simulink model "TwoCellAMM"  (R2016b)
settings: Solver=VariableStepAuto  StartTime=0.0  StopTime=50.0  RelTol=1e-3
undefined symbols (not defined in the file or in its folder): k1, k2, m1, m2
libraries: simulink x1
settings Model: Creator=a1630459  LastModifiedBy=a1630459

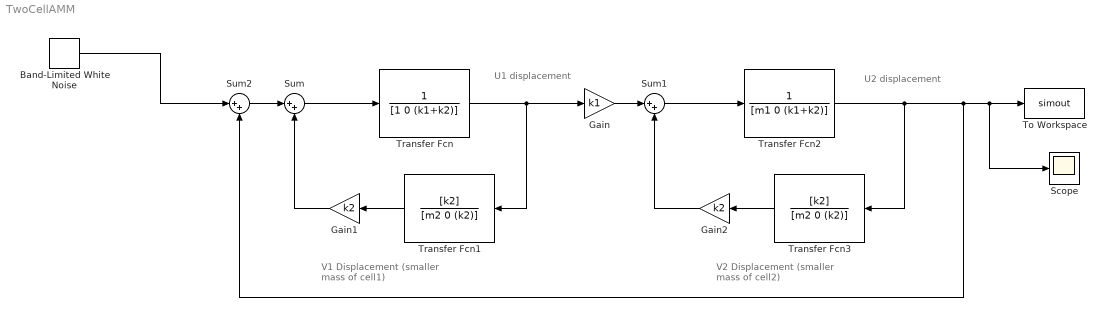
== system TwoCellAMM ==
  note: V1 Displacement
      | (smaller mass of cell1)
  note: U2 displacement
  note: U1 displacement
  note: V2 Displacement
      | (smaller mass of cell2)
  Band-Limited White Noise : simulink/Sources/Band-Limited White Noise  Cov=[0.1]  Ts=0.1  seed=[23341]
  Gain : Gain  Gain=k1
  Gain1 : Gain  Gain=k2
  Gain2 : Gain  Gain=k2
  Scope : Scope
  Sum : Sum  Inputs=|++
  Sum1 : Sum  Inputs=|++
  Sum2 : Sum  Inputs=|++
  To Workspace : ToWorkspace  VariableName=simout  SaveFormat=Timeseries  SampleTime=-1
  Transfer Fcn : TransferFcn  Denominator=[1 0 (k1+k2)]  ContinuousStateAttributes='displacement'
  Transfer Fcn1 : TransferFcn  Numerator=[k2]  Denominator=[m2 0 (k2)]  ContinuousStateAttributes='displacement'
  Transfer Fcn2 : TransferFcn  Denominator=[m1 0 (k1+k2)]  ContinuousStateAttributes='displacement'
  Transfer Fcn3 : TransferFcn  Numerator=[k2]  Denominator=[m2 0 (k2)]  ContinuousStateAttributes='displacement'
  wires:
  Sum/1 -> Transfer Fcn/1
  Gain/1 -> Sum1/1
  Transfer Fcn/1 -> Transfer Fcn1/1, Gain/1
  Transfer Fcn1/1 -> Gain1/1
  Gain1/1 -> Sum/2
  Sum2/1 -> Sum/1
  Sum1/1 -> Transfer Fcn2/1
  Gain2/1 -> Sum1/2
  Transfer Fcn3/1 -> Gain2/1
  Transfer Fcn2/1 -> Transfer Fcn3/1, Scope/1, To Workspace/1, Sum2/2
  Band-Limited White Noise/1 -> Sum2/1
